simulink model "smooth_simu"  (R2024a)
settings: Solver=FixedStepDiscrete  StartTime=0.0  StopTime=10.0  RelTol=1e-3
settings Model: Creator=Administrator  LastModifiedBy=Administrator
settings OptimizationCC: DefaultParameterBehavior=Inlined  EnhancedBackFolding=on  PassReuseOutputArgsAs=Individual arguments  ZeroExternalMemoryAtStartup=off  ZeroInternalMemoryAtStartup=off  OptimizeBlockOrder=speed  DifferentSizesBufferReuse=on  OptimizationCustomize=off  EfficientTunableParamExpr=on
settings DebuggingCC: ParameterTunabilityLossMsg=error
settings HardwareCC: ProdBitPerPointer=32  ProdBitPerSizeT=32  ProdBitPerPtrDiffT=32  ProdLargestAtomicInteger=Long  ProdLargestAtomicFloat=Double  ProdWordSize=32  ProdHWDeviceType=NXP->Cortex-M4
settings SFSimCC: MATLABDynamicMemAlloc=off
settings RTWCC: Description=Embedded Coder  SystemTargetFile=ert.tlc  TemplateMakefile=ert_default_tmf  GenerateReport=on  LaunchReport=on  TargetLang=C++
settings CodeAppCC: ForceParamTrailComments=on  IgnoreCustomStorageClasses=off  OperatorAnnotations=on  SimulinkDataObjDesc=on  SFDataObjDesc=on  InsertBlockDesc=on
settings ERTTargetCC: TargetLangStandard=C++11 (ISO)  GenerateSampleERTMain=on  CodeInterfacePackaging=C++ class  InlinedParameterPlacement=NonHierarchical  RootIOFormat=Structure reference  ERTCustomFileTemplate=example_file_process.tlc

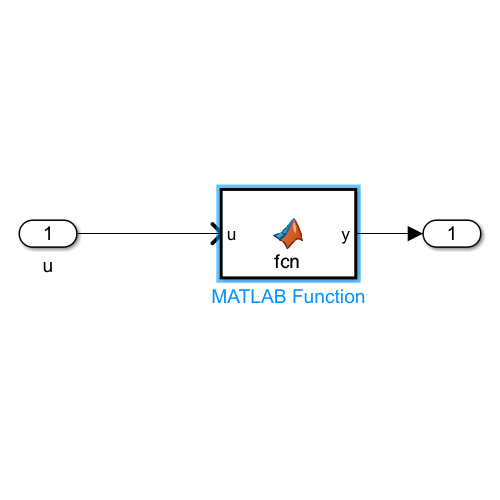
[thumbnail: Simulink's stored preview of the top-level diagram]
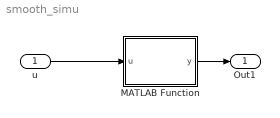
== system smooth_simu ==
  u : Inport  OutDataTypeStr=single  PortDimensions=[100,1]
  MATLAB Function : MATLAB Function  TreatAsAtomicUnit=on
  Out1 : Outport
  wires:
  MATLAB Function/1(y) -> Out1/1
  u/1 -> MATLAB Function/1(u)

== matlab function smooth_simu/MATLAB Function ==
  data: u input; y output
function y = fcn(u)
  
theSmoothDataRows=smoothdata(u,'gaussian',3);

Fs=25
Y=fft(theSmoothDataRows(:,:));
N=length(Y);
P2=abs(Y/N);
P1=P2(1:N/2+1);
P1(2:end-1)=2*P1(2:end-1);
 
f=(0:N-1)*Fs/N;
f=f(1:N/2+1);
plot(f,P1)
[maxValue,maxIndex]=max(P1)


 
k = 3;   
 
[sortedA, sortedIndices] = sort(P1, 'descend');
 
topKIndices = sortedIndices(1:k);

 
disp(topKIndices);
disp(f(topKIndices(2)))
heatBeatValue=60*f(topKIndices(2));
y = heatBeatValue;
end
